simulink model "altitudeTest"  (R2015a)
settings: Solver=ode45  StartTime=0.0  StopTime=240  FixedStep=0.0001  RelTol=1e-3
values from neighbouring files (symbols this model uses):
  maxPitch = 20    [initSimulation.m]
libraries: simulink x2
settings Model: Creator=Ludger Heide  LastModifiedBy=Ludger Heide

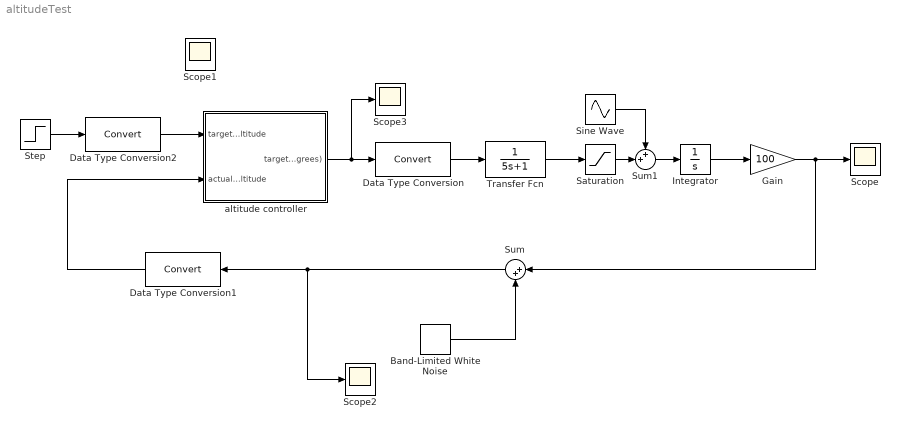
== system altitudeTest ==
  Band-Limited White Noise : simulink/Sources/Band-Limited White Noise  Cov=[100]  Ts=1/10  seed=[2123123123141]
  Data Type Conversion : DataTypeConversion
  Data Type Conversion1 : DataTypeConversion
  Data Type Conversion2 : DataTypeConversion
  Gain : Gain  Gain=100
  Integrator : Integrator
  Saturation : Saturate  UpperLimit=2  LowerLimit=-2
  Scope{,1..3} (4 alike) : Scope
      Scope2 settings: SaveName=ScopeData2
      Scope3 settings: SaveName=ScopeData3
  Sine Wave : Sin  Amplitude=0.5  Frequency=0.1  SampleTime=0
  Step : Step  After=10000  SampleTime=0
  Sum : Sum  Inputs=|++
  Sum1 : Sum  Inputs=++|
  Transfer Fcn : TransferFcn  Denominator=[5 1]
  altitude controller : Subsystem
  wires:
  Transfer Fcn/1 -> Saturation/1
  Integrator/1 -> Gain/1
  Data Type Conversion/1 -> Transfer Fcn/1
  Gain/1 -> Sum/1, Scope/1
  Data Type Conversion1/1 -> altitude controller/2(actualAltitude)
  Step/1 -> Data Type Conversion2/1
  Data Type Conversion2/1 -> altitude controller/1(targetAltitude)
  Band-Limited White Noise/1 -> Sum/2
  Saturation/1 -> Sum1/2
  Sum1/1 -> Integrator/1
  Sine Wave/1 -> Sum1/1
  Sum/1 -> Scope2/1, Data Type Conversion1/1
  altitude controller/1(targetPitch (degrees)) -> Scope3/1, Data Type Conversion/1

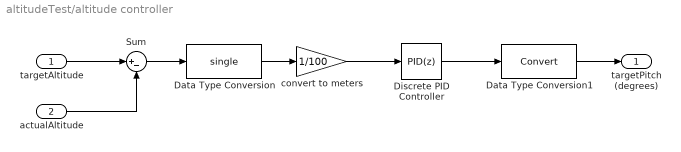
== system altitudeTest/altitude controller ==
  targetAltitude : Inport  OutDataTypeStr=int32
  actualAltitude : Inport  Port=2  OutDataTypeStr=int32
  Data Type Conversion : DataTypeConversion  OutMin=-1000  OutMax=100000  OutDataTypeStr=single
  Data Type Conversion1 : DataTypeConversion
  Discrete PID Controller : simulink/Continuous/PID Controller  Controller=PID  TimeDomain=Discrete-time  SampleTime=0.05  IntegratorMethod=Forward Euler  FilterMethod=Forward Euler  Form=Parallel  UseFilter=on  ControllerParametersSource=internal  P=0.470803059371346  I=0.024274424158626  D=1.80284909658714  N=1.40744934071441  InitialConditionSource=internal  InitialConditionForIntegrator=0  InitialConditionForFilter=0  ExternalReset=none  LimitOutput=on  UpperSaturationLimit=maxPitch  LowerSaturationLimit=-maxPitch  LinearizeAsGain=off  AntiWindupMode=clamping  Kb=1  TrackingMode=off  Kt=1  PParamMin=[]  PParamMax=[]  IParamMin=[]  IParamMax=[]  DParamMin=[]  DParamMax=[]  NParamMin=[]  NParamMax=[]  KbParamMin=[]  KbParamMax=[]  KtParamMin=[]  KtParamMax=[]  POutMin=[]  POutMax=[]  IOutMin=[]  IOutMax=[]  DOutMin=[]  DOutMax=[]  NOutMin=[]  NOutMax=[]  KbOutMin=[]  KbOutMax=[]  KtOutMin=[]  KtOutMax=[]  IntegratorOutMin=[]  IntegratorOutMax=[]  FilterOutMin=[]  FilterOutMax=[]  SumOutMin=[]  SumOutMax=[]  SumI1OutMin=[]  SumI1OutMax=[]  SumI2OutMin=[]  SumI2OutMax=[]  SumI3OutMin=[]  SumI3OutMax=[]  SumDOutMin=[]  SumDOutMax=[]  SaturationOutMin=[]  SaturationOutMax=[]  IntegratorContinuousStateAttributes=''  IntegratorStateMustResolveToSignalObject=off  IntegratorRTWStateStorageClass=Auto  FilterContinuousStateAttributes=''  FilterStateMustResolveToSignalObject=off  FilterRTWStateStorageClass=Auto  DifferentiatorICPrevScaledInput=0  DifferentiatorOutMin=[]  DifferentiatorOutMax=[]
  Sum : Sum  Inputs=|+-
  convert to meters : Gain  Gain=1/100
  targetPitch (degrees) : Outport  OutDataTypeStr=int8
  wires:
  targetAltitude/1 -> Sum/1
  actualAltitude/1 -> Sum/2
  Sum/1 -> Data Type Conversion/1
  Data Type Conversion/1 -> convert to meters/1
  Data Type Conversion1/1 -> targetPitch (degrees)/1
  convert to meters/1 -> Discrete PID Controller/1
  Discrete PID Controller/1 -> Data Type Conversion1/1
